simulink model "sih26038_screening_workflow_v9_0"  (R2026a)
settings: Solver=FixedStepDiscrete  StopTime=simulation_hours*3600  FixedStep=step_seconds
values from neighbouring files (symbols this model uses):
  acquisition_rate = 10.0    (= 10)    [build_sih26038_simulink_v9_0.m]
  auto_screen_fraction = 0.3356    [build_sih26038_simulink_v9_0.m]
  bandwidth_mbps = 20    [build_sih26038_simulink_v9_0.m]
  human_review_fraction = 0.2401    [build_sih26038_simulink_v9_0.m]
  image_mb = 2.5    [build_sih26038_simulink_v9_0.m]
  mid_capacity = 20    [build_sih26038_simulink_v9_0.m]
  mid_pool = 4    [build_sih26038_simulink_v9_0.m]
  recapture_fraction = 0.0    (= 0)    [build_sih26038_simulink_v9_0.m]
  recapture_service = 5    [build_sih26038_simulink_v9_0.m]
  refer_capacity = 15    [build_sih26038_simulink_v9_0.m]
  refer_fraction = 0.4243    [build_sih26038_simulink_v9_0.m]
  refer_pool = 2    [build_sih26038_simulink_v9_0.m]
  step_seconds = 60    [build_sih26038_simulink_v9_0.m]
settings Model: Creator=aersews  LastModifiedBy=aersews

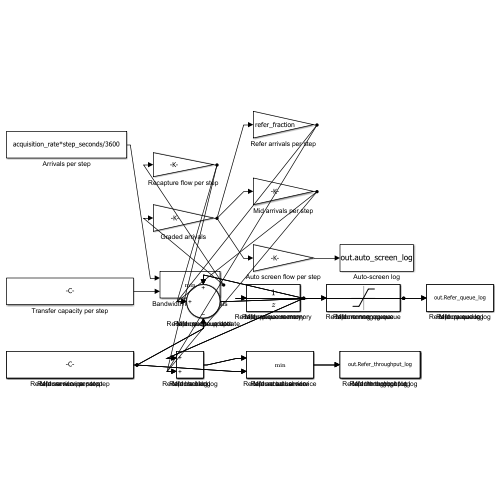
[thumbnail: Simulink's stored preview of the top-level diagram]
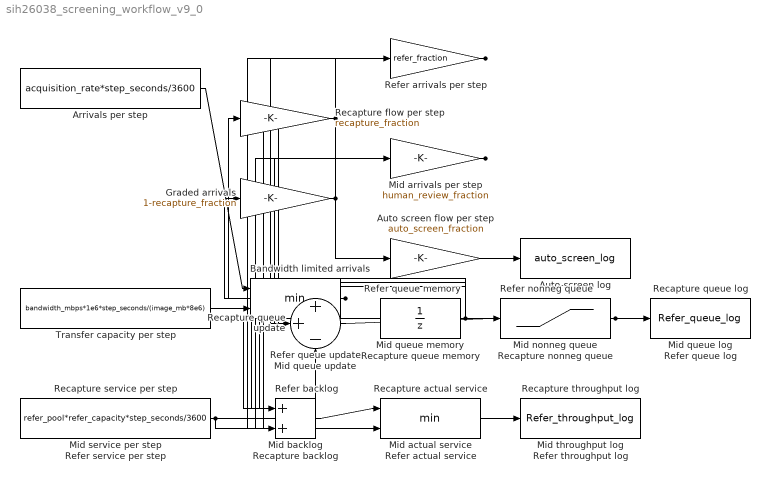
== system sih26038_screening_workflow_v9_0 ==
  Arrivals per step : Constant  Value=acquisition_rate*step_seconds/3600
  Auto screen flow per step : Gain  Gain=auto_screen_fraction
  Auto-screen log : ToWorkspace  VariableName=auto_screen_log  SaveFormat=Timeseries  SampleTime=step_seconds
  Bandwidth limited arrivals : MinMax  Inputs=2
  Graded arrivals : Gain  Gain=1-recapture_fraction
  Mid actual service : MinMax  Inputs=2
  Mid arrivals per step : Gain  Gain=human_review_fraction
  Mid backlog : Sum
  Mid nonneg queue : Saturate  UpperLimit=1e6  LowerLimit=0
  Mid queue log : ToWorkspace  VariableName=Mid_queue_log  SaveFormat=Timeseries  SampleTime=step_seconds
  Mid queue memory : UnitDelay  SampleTime=step_seconds
  Mid queue update : Sum  Inputs=++-
  Mid service per step : Constant  Value=mid_pool*mid_capacity*step_seconds/3600
  Mid throughput log : ToWorkspace  VariableName=Mid_throughput_log  SaveFormat=Timeseries  SampleTime=step_seconds
  Recapture actual service : MinMax  Inputs=2
  Recapture backlog : Sum
  Recapture flow per step : Gain  Gain=recapture_fraction
  Recapture nonneg queue : Saturate  UpperLimit=1e6  LowerLimit=0
  Recapture queue log : ToWorkspace  VariableName=Recapture_queue_log  SaveFormat=Timeseries  SampleTime=step_seconds
  Recapture queue memory : UnitDelay  SampleTime=step_seconds
  Recapture queue update : Sum  Inputs=++-
  Recapture service per step : Constant  Value=recapture_service*step_seconds/3600
  Recapture throughput log : ToWorkspace  VariableName=Recapture_throughput_log  SaveFormat=Timeseries  SampleTime=step_seconds
  Refer actual service : MinMax  Inputs=2
  Refer arrivals per step : Gain  Gain=refer_fraction
  Refer backlog : Sum
  Refer nonneg queue : Saturate  UpperLimit=1e6  LowerLimit=0
  Refer queue log : ToWorkspace  VariableName=Refer_queue_log  SaveFormat=Timeseries  SampleTime=step_seconds
  Refer queue memory : UnitDelay  SampleTime=step_seconds
  Refer queue update : Sum  Inputs=++-
  Refer service per step : Constant  Value=refer_pool*refer_capacity*step_seconds/3600
  Refer throughput log : ToWorkspace  VariableName=Refer_throughput_log  SaveFormat=Timeseries  SampleTime=step_seconds
  Transfer capacity per step : Constant  Value=bandwidth_mbps*1e6*step_seconds/(image_mb*8e6)
  wires:
  Recapture flow per step/1 -> Recapture queue update/2, Recapture backlog/2
  Recapture service per step/1 -> Recapture queue update/3, Recapture actual service/2
  Recapture queue memory/1 -> Recapture queue update/1, Recapture backlog/1
  Recapture queue update/1 -> Recapture nonneg queue/1
  Recapture nonneg queue/1 -> Recapture queue memory/1, Recapture queue log/1
  Recapture backlog/1 -> Recapture actual service/1
  Recapture actual service/1 -> Recapture throughput log/1
  Mid arrivals per step/1 -> Mid queue update/2, Mid backlog/2
  Mid service per step/1 -> Mid queue update/3, Mid actual service/2
  Mid queue memory/1 -> Mid queue update/1, Mid backlog/1
  Mid queue update/1 -> Mid nonneg queue/1
  Mid nonneg queue/1 -> Mid queue memory/1, Mid queue log/1
  Mid backlog/1 -> Mid actual service/1
  Mid actual service/1 -> Mid throughput log/1
  Refer arrivals per step/1 -> Refer queue update/2, Refer backlog/2
  Refer service per step/1 -> Refer queue update/3, Refer actual service/2
  Refer queue memory/1 -> Refer queue update/1, Refer backlog/1
  Refer queue update/1 -> Refer nonneg queue/1
  Refer nonneg queue/1 -> Refer queue memory/1, Refer queue log/1
  Refer backlog/1 -> Refer actual service/1
  Refer actual service/1 -> Refer throughput log/1
  Arrivals per step/1 -> Bandwidth limited arrivals/1
  Transfer capacity per step/1 -> Bandwidth limited arrivals/2
  Bandwidth limited arrivals/1 -> Recapture flow per step/1, Graded arrivals/1
  Graded arrivals/1 -> Mid arrivals per step/1, Refer arrivals per step/1, Auto screen flow per step/1
  Auto screen flow per step/1 -> Auto-screen log/1
